simulink model "Example_1"  (R2017b)
settings: Solver=VariableStepAuto  StartTime=0.0  StopTime=20  RelTol=1e-3
settings Model: Creator=hoang  LastModifiedBy=hoang

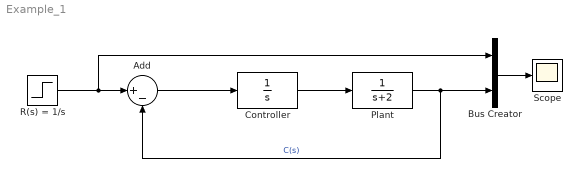
== system Example_1 ==
  Add : Sum  Inputs=|+-
  Bus Creator : BusCreator  Inputs=2
  Controller : TransferFcn  Denominator=[1 0]
  Plant : TransferFcn  Denominator=[1 2]
  R(s) = 1/s : Step  Time=5  SampleTime=0
  Scope : Scope
  wires:
  Controller/1 -> Plant/1
  Add/1 -> Controller/1
  Plant/1 -> Bus Creator/2, Add/2  "C(s)"
  R(s) = 1/s/1 -> Bus Creator/1, Add/1
  Bus Creator/1 -> Scope/1
